simulink model "Final_project"  (R2015b)
settings: Solver=FixedStepDiscrete  StartTime=0.0  StopTime=10.0  RelTol=1e-3
InitFcn:
  | parameters
values from neighbouring files (symbols this model uses):
  Ak = 100    [parameters.m]
  b = 100    [parameters.m]
  dT = 0.01    [parameters.m]
  H = 20    [parameters.m]
  m = 2000    [parameters.m]
  pot_gain = .33    (= 0.33)    [parameters.m]
  pot_offset = 512    [parameters.m]
  R = 1/5    (= 0.2)    [parameters.m]
  V_Ki = 50    [parameters.m]
  V_Kp = 5000    [parameters.m]
undefined symbols (not defined in the file or in its folder): A10, A13, A14, AN0, AN12, B, B13, B4, B6, C6, D, D11, D4, DiscIntNeverNeededParam, F17, F3, F4, G4, H4, L3, PA10, PA11, PA12, PA13, PA14, PA5, PA6, PA7, PA8, PA9, PB10, PB7, PC6, PD10, PD11, PG4, R10, R16, R5, R8, T15
libraries: Conv_Lib x54, rappid_564xl_ec_toolbox x34, Veh_Sim x9, simulink x4, U_of_M_5643_blockset x1
(part 1 of 2)
settings Model: Creator=raoulkumar  LastModifiedBy=sutorimb
settings DataIOCC: ExternalInput=off  InitialState=off  SaveOutput=off  SignalLogging=off  SaveTime=off
settings OptimizationCC: DefaultParameterBehavior=Inlined  OptimizeModelRefInitCode=on  LifeSpan=1
settings DebuggingCC: InheritedTsInSrcMsg=none  SingleTaskRateTransMsg=error  UnconnectedInputMsg=error  UnconnectedOutputMsg=error  UnconnectedLineMsg=error  UnknownTsInhSupMsg=error
settings HardwareCC: ProdBitPerPointer=32  ProdLargestAtomicInteger=Long  ProdLargestAtomicFloat=Double  ProdEndianess=BigEndian  ProdWordSize=32  ProdHWDeviceType=Freescale->32-bit PowerPC
settings RTWCC: SystemTargetFile=rappid564xl.tlc  MakeCommand=rappid_564xl_make_rtw  TemplateMakefile=rappid_564xl_default_tmf  PostCodeGenCommand=rappid_analyzegencode(buildInfo)  Description=RAppID Toolbox MPC564xL Code Generation Target (rappid)  GenerateReport=on  IncludeHyperlinkInReport=on  LaunchReport=on  GenerateTraceReport=on  GenerateTraceReportSl=on  GenerateTraceReportSf=on  GenerateTraceReportEml=on
settings CodeAppCC: IgnoreCustomStorageClasses=off
settings STFCustomTargetCC: ConcurrentExecutionCompliant=off  GeneratePreprocessorConditionals=Use local settings  CombineOutputUpdateFcns=on  SuppressErrorStatus=on  ERTCustomFileBanners=on  SupportContinuousTime=off  SupportNonInlinedSFcns=off  MATLABClassNameForMDSCustomization=Simulink.SoftwareTarget.ERTCustomization  CPPClassGenCompliant=off  GRTInterface=off  SystemTargetFile=rappid564xl.tlc
settings ERTTargetCC: ParMdlRefBuildCompliant=off  CompOptLevelCompliant=off  ConcurrentExecutionCompliant=off  SuppressErrorStatus=on  ERTFirstTimeCompliant=off  ModelStepFunctionPrototypeControlCompliant=off  CPPClassGenCompliant=off  UseToolchainInfoCompliant=off  InlinedParameterPlacement=NonHierarchical  ERTCustomFileTemplate=example_file_process.tlc

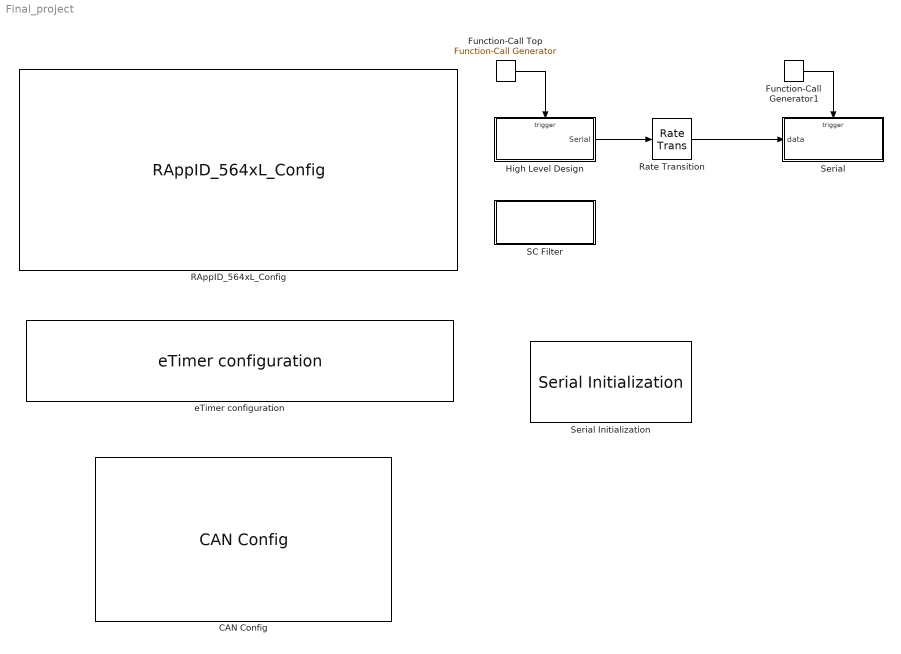
== system Final_project ==
  CAN Config : rappid_564xl_ec_toolbox/MPC564xL/Communication Blocks/CAN Config  Priority=1  can_unit=A  can_unit_v2=0  can_idam=A - One full ID (standard or extended) per filter element.  can_srx_dis=1 - Self reception disabled  can_presdiv=4  can_rjw=3  can_pseg1=5  can_pseg2=5  can_clk_src=0 - The CAN engine clock source is the oscillator clock  can_lpb=0 - Loop Back disabled  can_smp=0 - One sample is used to determine the bit value  can_boff_rec=0 - Automatic recovering from Bus Off state enabled  can_tsyn=0 - Timer Sync feature disabled  can_lbuf=0 - Buffer with highest priority is transmitted first  can_lom=0 - Listen Only Mode is deactivated  can_propseg=2
  Function-Call Generator1 : simulink/Ports & Subsystems/Function-Call Generator  sample_time=0.05  numberOfIterations=1
  Function-Call Top : simulink/Ports & Subsystems/Function-Call Generator  sample_time=dT  numberOfIterations=1
  High Level Design : Subsystem  TreatAsAtomicUnit=on
  RAppID_564xL_Config : rappid_564xl_ec_toolbox/MPC564xL/RAppID_564xL_Config  SystemClock=120  XTAL=40  MC_clock_60=12  MC_clock_80=16  MC_clock_120=10  SWG_clock_60=20  SWG_clock_80=13.334  SWG_clock_120=20  Compiler=CodeWarrior  MemTarget=FLASH  Part=MPC5643L  Package=144 LQFP  global_int_priority=10  base_tick_priority=11  sys_task_supress=off  exception_handlers=off  stored_mdl_name=Final_project  freemaster_interface=Oops  freemaster_rx_pin="LINFlex_0 Rx Pin 116 : \"PB[3]\""  freemaster_tx_pin="LINFlex_0 Tx Pin 114 : \"PB[2]\""  freemaster_interface_1=Serial 0  freemaster_enable=on  freemaster_rate=115200  freemaster_tx0_pin=18 : B[2] : 114 : A14  freemaster_rx0_pin=19 : B[3] : 116 : B13  freemaster_tx1_pin=57 : D[9] : 26 : L3  freemaster_rx1_pin=29 : B[13] : 60 : R10  freemaster_can_channel=1CH  freemater_can_speed=500K  freemaster_can_msgig=0x7AA  ccp_interface=None  ccp_enable=off  ccp_can_channel=CH1 (MB 0 - 1)  ccp_can_speed=500K  ccp_can_cro_id=256  ccp_can_dto_id=257  ccp_dev_id=RappID  ccp_dev_addr=0  ccp_odt=3  ccp_daq=3  pil_enable=off  pil_bam=off  comport=4  pil_rate=115200  bam_password_def=on  bam_password=0xFEEDFACECAFEBEEF  bam_sa_cs=off  bam_start_address=0x0  bam_code_size=0x7000  cons_dspi=on  cons_can=on  cons_adc=on  cons_pwm=on  cons_ctu=on  cons_swg=on  cons_eTimer=on  cons_fm=on
  Rate Transition : RateTransition
  SC Filter : Subsystem
  Serial : Subsystem  TreatAsAtomicUnit=on
  Serial Initialization : U_of_M_5643_blockset/Serial/Serial Initialization
  eTimer configuration : rappid_564xl_ec_toolbox/MPC564xL/Motor Control Blocks/eTimer configuration  SubModule=0  TimerChan=0  subMod=0  channel=0  CountMode=100 - Quadrature count mode using primary and secondary sources  CNTMODE=4  CountOnce=0 - Count repeatedly  ONCE=0  CountLength=0 - Continue counting to roll over  LENGTH=0  CountDirection=0 - Count up  DIR=0  OutputEnable=0 - The external pin is configured as an input  OEN=0  CoChanInit=00 - Other channels cannot force re-initialization of this channel  COINIT=0  StopAction=0 - Output enable is unaffected by stop mode  STPEN=0  ReloadOnCapt=00 - Do not reload the counter on a capture event  ROC=0  PrimarySource=00000 - Counter #0 input pin  PRISRC=0  PrimSrcPol=0 - True polarity  PIPS=0  SecondarySource=00001 - Counter #1 input pin  SECSRC=1  SecSrcPol=0 - True polarity  SIPS=0  FILT_CNT=0  FILT_PER=0  FILT=0  OutputMode=0000 - Software controlled  OUTMODE=0  OutputPol=0 - True polarity  OPS=0  MasterMode=0 - Disable broadcast of this channel output  MSTR=0  ForcedOutVal=0  VAL=0  CoForce=0 - Other channels cannot force this channel output  COFRC=0  CompLoad1=000 - COMP1 is never preload  CLC1=0  CompLoad2=000 - COMP2 is never preload  CLC2=0  CompareMode="00 - COMP1 and COMP2  are used when the counter is counting up"  CMPMODE=0  CaptMode1=00 - Capture disabled  CPT1MODE=0  CaptMode2=00 - Capture disabled  CPT2MODE=0  OneShCaptMode=0 - Free running mode is selected  ONESHOT=0  CaptFIFO=0  CFWM=0  CNTRinit=0  COMP1init=0  COMP2init=0  mod0ch0pin="0   : PA0  : [ 73 ] : [ T14 ]  input/output"  mod0ch1pin="1   : PA1  : [ 74 ] : [ R14 ]  input/output"  mod0ch2pin=None  mod0ch3pin=None  mod0ch4pin=None  mod0ch5pin=None  mod1ch0pin=None  mod1ch1pin=None  mod1ch2pin=None  mod1ch3pin=None  mod1ch4pin=None  mod1ch5pin=None  mod2ch0pin=None  mod2ch1pin=None  mod2ch2pin=None  mod2ch3pin=None  mod2ch4pin=None  mod2ch5pin=None  pcrNum0=0  pcrNum1=1  pcrNum2=255  pcrNum3=255  pcrNum4=255  pcrNum5=255  TCFIE=off  TCF1IE=off  TCF2IE=off  TOFIE=off  IELFIE=off  IEHFIE=off  ICF1IE=off  ICF2IE=off  INTDMA=0
  wires:
  Function-Call Top/1 -> High Level Design/Trigger
  Function-Call Generator1/1 -> Serial/Trigger
  High Level Design/1(Serial) -> Rate Transition/1
  Rate Transition/1 -> Serial/1(data)

== system Final_project/High Level Design ==
  function : TriggerPort  TriggerType=function-call
  "\tVehicle Model" : Subsystem
  Automatic Cruise Control : Subsystem
  Automatic Steering : Subsystem
  Delay : Delay  DelayLength=1  InitialCondition=0
  Inputs : Subsystem
  Outputs : Subsystem
  Terminator : Terminator
  Serial : Outport
  wires:
  Outputs/1("x, y, pxi (Cars 1-6)") -> Serial/1
  Inputs/3(Cruise Control Speed) -> Automatic Cruise Control/1(Cruise Control Speed)
  "\tVehicle Model"/1(s,n,psi us (This Car)) -> Automatic Steering/3("s, n, psi, us (This Car)"), Delay/1, Outputs/2("s, n, psi, us (This Car)")
  Inputs/2(ACC_enable) -> Automatic Cruise Control/2(Acc Enable)
  Inputs/6(Automatic Steering Enable) -> Automatic Steering/1(Automatic Steering Enable)
  Inputs/4(Steering Angle (delta)) -> "\tVehicle Model"/2(steering angle (delta)), Automatic Steering/2(Steering Angle (delta))
  Inputs/5(Throttle (Fd)) -> Automatic Cruise Control/5(Fd)
  "\tVehicle Model"/2(Self-Aligning Torque) -> Outputs/4(Self-Aligning Torque)
  Inputs/1("s, n, psi, us (Cars 1-6)") -> Automatic Cruise Control/3("s, n, psi, us (Cars 1-6)"), Outputs/1("s, n, psi, us (Cars 1-6)")
  "\tVehicle Model"/3(u) -> Outputs/3(u (This car))
  Automatic Steering/1(Auto Torque) -> Outputs/5(Auto Torque)
  Automatic Cruise Control/1(Fd_out) -> "\tVehicle Model"/1(Fd)
  Delay/1 -> Automatic Cruise Control/4(s,n,psi,us (This Car))
  Automatic Steering/2(delta_desired) -> Terminator/1

== system Final_project/SC Filter ==
  Constant1 : Constant  Value=1e6  OutDataTypeStr=uint32
  Constant2 : Constant  Value=0  OutDataTypeStr=uint32
  Constant3 : Constant  Value=50  OutDataTypeStr=uint32
  Simple PWM Output : rappid_564xl_ec_toolbox/MPC564xL/Motor Control Blocks/Simple PWM Output  Priority=1  pwmModule=0  pwmMod=0  SubModule=1  subMod=1  InitFreq=1000000  resolution=1 %  resValue=1  InitDutyA=0  InitDutyB=50  align=A B - edge aligned  PhaseShift_A=0  PhaseShift=0  Phase_A=0  Phase_B=0  centered=0  DoubleS=off  doubleSw=off  debugSw=off  debug_mode=0  pin_A0=None  pin_B0=None  pin_X0=None  pin_A1=None  pin_B1="38  : PC6  : [ 142 ] : [ D4 ]"  pin_X1=None  pin_A2=None  pin_B2=None  pin_X2=None  pin_A3=None  pin_B3=None  pin_X3=None  pin1_A0=None  pin1_B0=None  pin1_X0=None  pin1_A1=None  pin1_B1=None  pin1_X1=None  pin1_A2=None  pin1_B2=None  pin1_X2=None  pin1_A3=None  pin1_B3=None  pin1_X3=None  pcrNumA=255  pcrNumB=38  pcrNumX=255  polA=off  polB=off  polX=off  octrl=0  syncFrom0=off  masterSync=0  outVal0=off  outVal1=off  outVal2=off  outVal3=off  outVal4=on  outVal5=on  outTrig=48
  wires:
  Constant1/1 -> Simple PWM Output/1
  Constant2/1 -> Simple PWM Output/2
  Constant3/1 -> Simple PWM Output/3

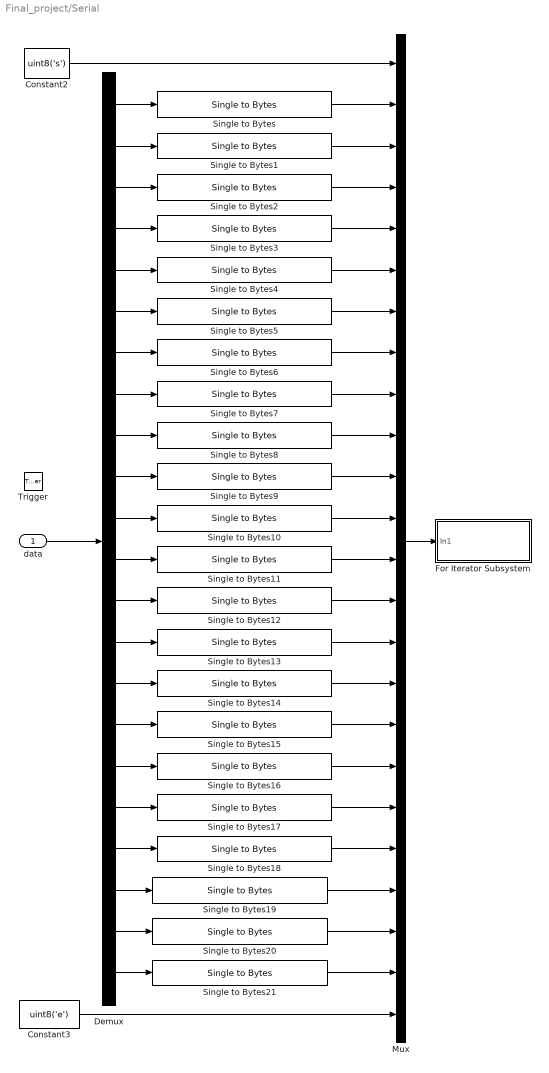
== system Final_project/Serial ==
  data : Inport
  Trigger : TriggerPort  TriggerType=function-call
  Constant2 : Constant  Value=uint8('s')  OutDataTypeStr=uint8
  Constant3 : Constant  Value=uint8('e')  OutDataTypeStr=uint8
  Demux : Demux  Outputs=22
  For Iterator Subsystem : Subsystem
  Mux : Mux  Inputs=24
  Single to Bytes{,1..21} (22 alike) : Conv_Lib/Single to Bytes
  wires:
  Constant2/1 -> Mux/1
  Single to Bytes/1 -> Mux/2
  Single to Bytes1/1 -> Mux/3
  Single to Bytes2/1 -> Mux/4
  Single to Bytes3/1 -> Mux/5
  Single to Bytes4/1 -> Mux/6
  Single to Bytes5/1 -> Mux/7
  Single to Bytes6/1 -> Mux/8
  Single to Bytes7/1 -> Mux/9
  Single to Bytes8/1 -> Mux/10
  Single to Bytes9/1 -> Mux/11
  Single to Bytes10/1 -> Mux/12
  Single to Bytes11/1 -> Mux/13
  Single to Bytes12/1 -> Mux/14
  Single to Bytes13/1 -> Mux/15
  Single to Bytes15/1 -> Mux/17
  Single to Bytes16/1 -> Mux/18
  Single to Bytes17/1 -> Mux/19
  Mux/1 -> For Iterator Subsystem/1(In1)
  Demux/1 -> Single to Bytes/1
  Demux/2 -> Single to Bytes1/1
  Demux/3 -> Single to Bytes2/1
  Demux/4 -> Single to Bytes3/1
  Demux/5 -> Single to Bytes4/1
  Demux/6 -> Single to Bytes5/1
  Demux/7 -> Single to Bytes6/1
  Demux/8 -> Single to Bytes7/1
  Demux/9 -> Single to Bytes8/1
  Demux/10 -> Single to Bytes9/1
  Demux/11 -> Single to Bytes10/1
  Demux/12 -> Single to Bytes11/1
  Demux/13 -> Single to Bytes12/1
  Demux/14 -> Single to Bytes13/1
  Demux/15 -> Single to Bytes14/1
  Demux/16 -> Single to Bytes15/1
  Demux/17 -> Single to Bytes16/1
  Demux/18 -> Single to Bytes17/1
  data/1 -> Demux/1
  Single to Bytes14/1 -> Mux/16
  Demux/19 -> Single to Bytes18/1
  Demux/20 -> Single to Bytes19/1
  Demux/21 -> Single to Bytes20/1
  Demux/22 -> Single to Bytes21/1
  Single to Bytes18/1 -> Mux/20
  Single to Bytes19/1 -> Mux/21
  Single to Bytes20/1 -> Mux/22
  Single to Bytes21/1 -> Mux/23
  Constant3/1 -> Mux/24

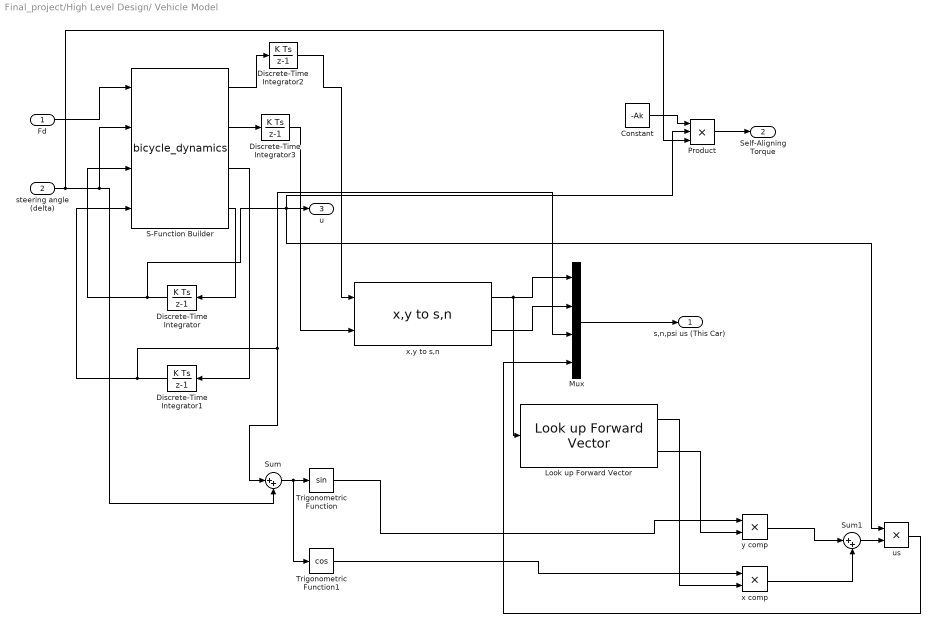
== system Final_project/High Level Design/	Vehicle Model ==
  Fd : Inport
  steering angle (delta) : Inport  Port=2
  Constant : Constant  Value=-Ak  OutDataTypeStr=single
  Discrete-Time Integrator{,1..3} (4 alike) : DiscreteIntegrator  SampleTime=-1  ICPrevOutput=DiscIntNeverNeededParam  ICPrevScaledInput=DiscIntNeverNeededParam
  Look up Forward Vector : Veh_Sim/Look up Forward Vector  SystemSampleTime=-1
  Mux : Mux
  Product : Product  Inputs=3
  S-Function Builder : S-Function  InitFcn=try, set_param(gcb,'FunctionName','bicycle_dynamics'), end  FunctionName=bicycle_dynamics  SFunctionModules=bicycle_dynamics_wrapper  SFunctionDeploymentMode=off  EnableBusSupport=off  mask(S-Function Builder){}
      mask help: Simulink:masks:SFunctionBuilder_MD
      mask init:
      | val = [[.9  0.75 0.75 1 1 .9 .9 1]',[1 1 0.75 0.75 .9 .9 1 .9]'];try , sys = get_param(gcb,'SfunBuilderFcnName');if isempty(sys), sys = get_param(gcb,'FunctionName'); end,catch, sys = get_param(gcb,'FunctionName'); end
      settings: CopyFcn=set_param(gcbh,'LinkStatus','none')  PreSaveFcn=try, set_param(gcb,'FunctionName','bicycle_dynamics'), end  OpenFcn=sfunctionwizard(gcbh)
      mask Display: plot(val(:,1),val(:,2)),disp(sys), port_label('input',1,'Fd'), port_label('input',2,'delta'), port_label('input',3,'u'), port_label('input',4,'psi'), port_label('output',1,'x_dot'), port_label('output',2,'y_dot'), port_label('output',3,'psi_dot'), port_label('output',4,'u_dot')
  Sum : Sum  Inputs=|++
  Sum1 : Sum  Inputs=|++
  Trigonometric Function : Trigonometry
  Trigonometric Function1 : Trigonometry  Operator=cos
  "us " : Product
  x comp : Product
  x,y to s,n : Veh_Sim/x,y to s,n  SystemSampleTime=-1
  y comp : Product
  s,n,psi us (This Car) : Outport
  Self-Aligning Torque : Outport  Port=2
  u : Outport  Port=3
  wires:
  Fd/1 -> S-Function Builder/1
  steering angle (delta)/1 -> Product/3, Sum/2, S-Function Builder/2
  S-Function Builder/4 -> Discrete-Time Integrator/1
  S-Function Builder/3 -> Discrete-Time Integrator1/1
  Discrete-Time Integrator/1 -> "us "/1, Product/2, u/1, S-Function Builder/3
  Discrete-Time Integrator1/1 -> Mux/3, Sum/1, S-Function Builder/4
  S-Function Builder/1 -> Discrete-Time Integrator2/1
  Discrete-Time Integrator2/1 -> x,y to s,n/1
  Discrete-Time Integrator3/1 -> x,y to s,n/2
  S-Function Builder/2 -> Discrete-Time Integrator3/1
  Constant/1 -> Product/1
  Product/1 -> Self-Aligning Torque/1
  Mux/1 -> s,n,psi us (This Car)/1
  x,y to s,n/1 -> Look up Forward Vector/1, Mux/1
  x,y to s,n/2 -> Mux/2
  Sum/1 -> Trigonometric Function1/1, Trigonometric Function/1
  Trigonometric Function/1 -> y comp/1
  Look up Forward Vector/2 -> y comp/2
  Trigonometric Function1/1 -> x comp/1
  Look up Forward Vector/1 -> x comp/2
  y comp/1 -> Sum1/1
  x comp/1 -> Sum1/2
  Sum1/1 -> "us "/2
  "us "/1 -> Mux/4

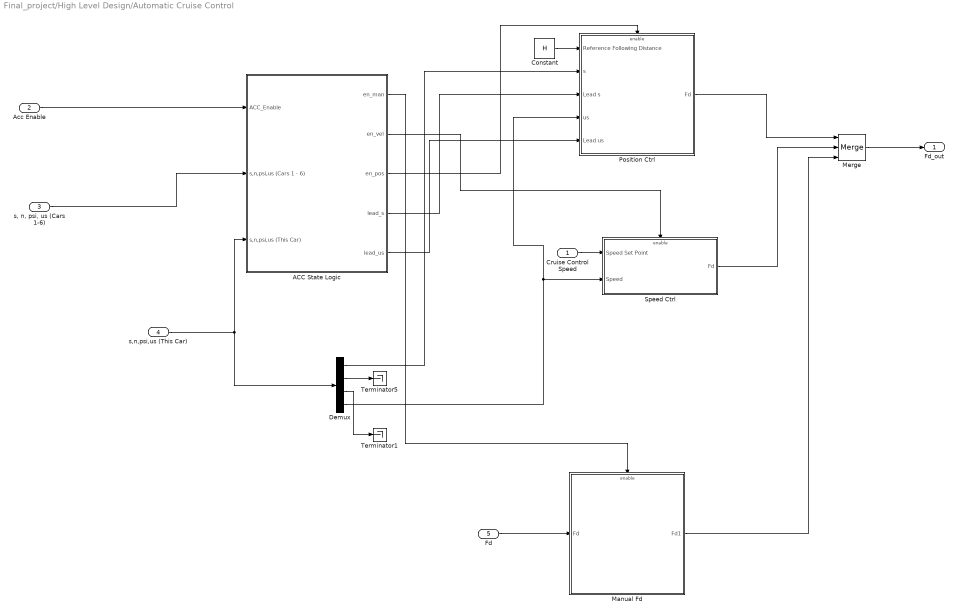
== system Final_project/High Level Design/Automatic Cruise Control ==
  Cruise Control Speed : Inport
  Acc Enable : Inport  Port=2
  "s, n, psi, us (Cars 1-6)" : Inport  Port=3
  s,n,psi,us (This Car) : Inport  Port=4
  Fd : Inport  Port=5
  ACC State Logic : Subsystem
  Constant : Constant  Value=H
  Demux : Demux
  Manual Fd : Subsystem  TreatAsAtomicUnit=on
  Merge : Merge  Inputs=3
  Position Ctrl : Subsystem  TreatAsAtomicUnit=on
  Speed Ctrl : Subsystem  TreatAsAtomicUnit=on
  Terminator1 : Terminator
  Terminator5 : Terminator
  Fd_out : Outport
  wires:
  Acc Enable/1 -> ACC State Logic/1(ACC_Enable)
  "s, n, psi, us (Cars 1-6)"/1 -> ACC State Logic/2(s,n,psi,us (Cars 1 - 6))
  s,n,psi,us (This Car)/1 -> Demux/1, ACC State Logic/3(s,n,psi,us (This Car))
  ACC State Logic/3(en_pos) -> Position Ctrl/Enable
  ACC State Logic/2(en_vel) -> Speed Ctrl/Enable
  ACC State Logic/4(lead_s) -> Position Ctrl/3(Lead s)
  Cruise Control Speed/1 -> Speed Ctrl/1(Speed Set Point)
  ACC State Logic/5(lead_us) -> Position Ctrl/5(Lead us)
  Demux/1 -> Position Ctrl/2(s)
  Demux/4 -> Position Ctrl/4(us), Speed Ctrl/2(Speed)
  Position Ctrl/1(Fd) -> Merge/1
  Speed Ctrl/1(Fd) -> Merge/2
  Constant/1 -> Position Ctrl/1(Reference Following Distance)
  Fd/1 -> Manual Fd/1(Fd)
  Manual Fd/1(Fd1) -> Merge/3
  ACC State Logic/1(en_man) -> Manual Fd/Enable
  Merge/1 -> Fd_out/1
  Demux/2 -> Terminator5/1
  Demux/3 -> Terminator1/1

== system Final_project/High Level Design/Automatic Steering ==
  Automatic Steering Enable : Inport
  Steering Angle (delta) : Inport  Port=2
  "s, n, psi, us (This Car)" : Inport  Port=3
  Constant : Constant  Value=0.5  OutDataTypeStr=single
  Controller : Subsystem  TreatAsAtomicUnit=on
  Demux : Demux
  Terminator : Terminator
  Terminator1 : Terminator
  Terminator3 : Terminator
  Auto Torque : Outport
  delta_desired : Outport  Port=2
  wires:
  Automatic Steering Enable/1 -> Controller/Enable
  Controller/1(Auto Torque) -> Auto Torque/1
  "s, n, psi, us (This Car)"/1 -> Demux/1
  Demux/4 -> Terminator/1
  Demux/3 -> Terminator1/1
  Demux/1 -> Terminator3/1
  Demux/2 -> Controller/1(n (This Car))
  Steering Angle (delta)/1 -> Controller/3(Delta (This Car))
  Constant/1 -> Controller/2(n desired)
  Controller/2(delta desired) -> delta_desired/1

== system Final_project/High Level Design/Inputs ==
  Digital Input : rappid_564xl_ec_toolbox/MPC564xL/General Purpose Blocks/Digital Input  gpio_outputs="13  : PA13 : [ 136 ] : [ C6 ]"  pinNum=[ 136 ]  pcrNum=13
  Digital Input1 : rappid_564xl_ec_toolbox/MPC564xL/General Purpose Blocks/Digital Input  gpio_outputs="14  : PA14 : [ 143 ] : [ B4 ]"  pinNum=[ 143 ]  pcrNum=14
  Gain : Gain  Gain=R/10
  Other Cars : Subsystem
  Select Speed (GPI 122-129) : Subsystem
  Throttle (Potentiometer) : Subsystem
  get wheel position : Subsystem
  "s, n, psi, us (Cars 1-6)" : Outport
  ACC_enable : Outport  Port=2
  Cruise Control Speed : Outport  Port=3
  Steering Angle (delta) : Outport  Port=4
  Throttle (Fd) : Outport  Port=5
  Automatic Steering Enable : Outport  Port=6
  wires:
  Other Cars/1("s, n, psi, us (Cars 1-6)") -> "s, n, psi, us (Cars 1-6)"/1
  Select Speed (GPI 122-129)/1(Speed) -> Cruise Control Speed/1
  get wheel position/1(Haptic Wheel Position (radians)) -> Gain/1
  Gain/1 -> Steering Angle (delta)/1
  Throttle (Potentiometer)/1(Fd) -> Throttle (Fd)/1
  Digital Input/1 -> ACC_enable/1
  Digital Input1/1 -> Automatic Steering Enable/1

== system Final_project/High Level Design/Outputs ==
  "s, n, psi, us (Cars 1-6)" : Inport
  "s, n, psi, us (This Car)" : Inport  Port=2
  u (This car) : Inport  Port=3
  Self-Aligning Torque : Inport  Port=4
  Auto Torque : Inport  Port=5
  Extract x,y,psi : Subsystem
  Extract x,y,psi (Cars 1 - 6) : Subsystem
  Mux : Mux  Inputs=3
  Output s,n,psi,us : Subsystem
  Sum1 : Sum  Inputs=|++
  write torque : Subsystem
  "x, y, pxi (Cars 1-6)" : Outport
  wires:
  Self-Aligning Torque/1 -> Sum1/1
  Auto Torque/1 -> Sum1/2
  Sum1/1 -> write torque/1(Reaction Torque)
  "s, n, psi, us (Cars 1-6)"/1 -> Extract x,y,psi (Cars 1 - 6)/1(s,n,psi,us (Cars 1 - 6))
  "s, n, psi, us (This Car)"/1 -> Output s,n,psi,us/1(s,n,psi.us), Extract x,y,psi/1(s,n,psi,us)
  Extract x,y,psi/1(x,y,psi) -> Mux/1
  Mux/1 -> "x, y, pxi (Cars 1-6)"/1
  u (This car)/1 -> Mux/2
  Extract x,y,psi (Cars 1 - 6)/1(x,y,psi (Cars 1 - 6)) -> Mux/3

== system Final_project/Serial/For Iterator Subsystem ==
  In1 : Inport
  Data Type Conversion : DataTypeConversion  OutDataTypeStr=uint8
  For Iterator : ForIterator  IterationLimit=90  IndexMode=Zero-based  IterationVariableDataType=int8
  Index Vector : MultiPortSwitch  DataPortOrder=Zero-based contiguous  Inputs=1  zeroidx=on
  S-Function : S-Function  FunctionName=SerialSend  SFunctionDeploymentMode=off  EnableBusSupport=off
      mask Display:
      | patch([0 0 1 1], [0 1 1 0], [255/255 255/255 0])
      | patch([0 0 0.05 0.05], [0 1 1 0], [0 0 255/255])
      | patch([1 1 0.95 0.95], [0 1 1 0], [0 0 255/255])
      | 
      | text (0.52, 0.8, ['Serial Send'], 'horizontalAlignment', 'center');
      | %text (0.5, .5, ['System Clock MHz: ' get_param(gcb,'SystemClock')], 'horizontalAlignment', 'center');
      | %text (0.5, .35, ['Baud Rate: ' get_param(gcb,'BaudRate')], 'horizontalAlignment', 'center');
      | text(0.5, 0.1, 'The University of Michigan', 'horizontalAlignment', 'center');
  wires:
  In1/1 -> Index Vector/2
  Index Vector/1 -> Data Type Conversion/1
  For Iterator/1 -> Index Vector/1
  Data Type Conversion/1 -> S-Function/1

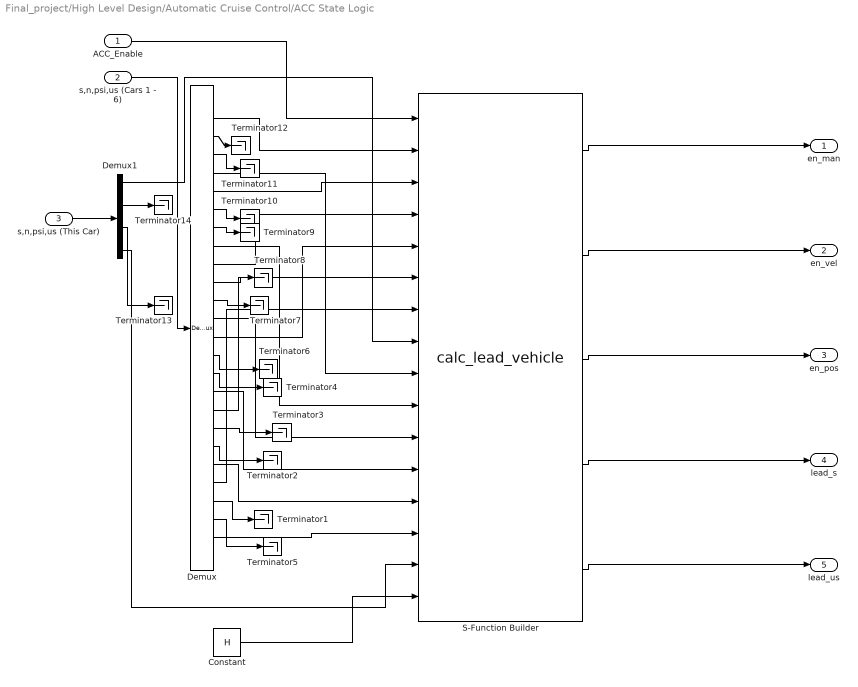
== system Final_project/High Level Design/Automatic Cruise Control/ACC State Logic ==
  ACC_Enable : Inport
  s,n,psi,us (Cars 1 - 6) : Inport  Port=2
  s,n,psi,us (This Car) : Inport  Port=3
  Constant : Constant  Value=H
  Demux : Demux  Outputs=24
  Demux1 : Demux
  S-Function Builder : S-Function  InitFcn=try, set_param(gcb,'FunctionName','calc_lead_vehicle'), end  FunctionName=calc_lead_vehicle  SFunctionModules=calc_lead_vehicle_wrapper  SFunctionDeploymentMode=off  EnableBusSupport=off  mask(S-Function Builder){}
      mask help: Simulink:masks:SFunctionBuilder_MD
      mask init: same as Final_project/High Level Design/	Vehicle Model/S-Function Builder
      settings: CopyFcn=set_param(gcbh,'LinkStatus','none')  PreSaveFcn=try, set_param(gcb,'FunctionName','calc_lead_vehicle'), end  OpenFcn=sfunctionwizard(gcbh)
      mask Display: plot(val(:,1),val(:,2)),disp(sys), port_label('input',1,'ACC_Enable'), port_label('input',2,'s1'), port_label('input',3,'s2'), port_label('input',4,'s3'), port_label('input',5,'s4'), port_label('input',6,'s5'), port_label('input',7,'s6'), port_label('input',8,'s'), port_label('input',9,'us1'), port_label('input',10,'us2'), port_label('input',11,'us3'), port_label('input',12,'us4'), port_label('input',13,'us5'), port_label('input',14,'us6'), port_label('input',15,'us'), port_label('input',16,'H'), port_label('output',1,'en_man'), port_label('output',2,'en_vel'), port_label('output',3,'en_pos'), port_label('output',4,'lead_s'), port_label('output',5,'lead_us')
  Terminator{1..14} (14 alike) : Terminator
  en_man : Outport
  en_vel : Outport  Port=2
  en_pos : Outport  Port=3
  lead_s : Outport  Port=4
  lead_us : Outport  Port=5
  wires:
  s,n,psi,us (Cars 1 - 6)/1 -> Demux/1
  s,n,psi,us (This Car)/1 -> Demux1/1
  ACC_Enable/1 -> S-Function Builder/1
  S-Function Builder/1 -> en_man/1
  S-Function Builder/2 -> en_vel/1
  S-Function Builder/3 -> en_pos/1
  S-Function Builder/4 -> lead_s/1
  S-Function Builder/5 -> lead_us/1
  Constant/1 -> S-Function Builder/16
  Demux1/4 -> S-Function Builder/15
  Demux/1 -> S-Function Builder/2
  Demux/4 -> S-Function Builder/9
  Demux/5 -> S-Function Builder/3
  Demux/8 -> S-Function Builder/10
  Demux/9 -> S-Function Builder/4
  Demux/12 -> S-Function Builder/11
  Demux/13 -> S-Function Builder/5
  Demux/16 -> S-Function Builder/12
  Demux/17 -> S-Function Builder/6
  Demux/20 -> S-Function Builder/13
  Demux/24 -> S-Function Builder/14
  Demux/21 -> S-Function Builder/7
  Demux1/1 -> S-Function Builder/8
  Demux/23 -> Terminator5/1
  Demux/22 -> Terminator1/1
  Demux/19 -> Terminator2/1
  Demux/18 -> Terminator3/1
  Demux/15 -> Terminator4/1
  Demux/14 -> Terminator6/1
  Demux/11 -> Terminator7/1
  Demux/10 -> Terminator8/1
  Demux/7 -> Terminator9/1
  Demux/6 -> Terminator10/1
  Demux/3 -> Terminator11/1
  Demux/2 -> Terminator12/1
  Demux1/3 -> Terminator13/1
  Demux1/2 -> Terminator14/1

== system Final_project/High Level Design/Automatic Cruise Control/Manual Fd ==
  Fd : Inport
  Enable : EnablePort
  Fd1 : Outport
  wires:
  Fd/1 -> Fd1/1

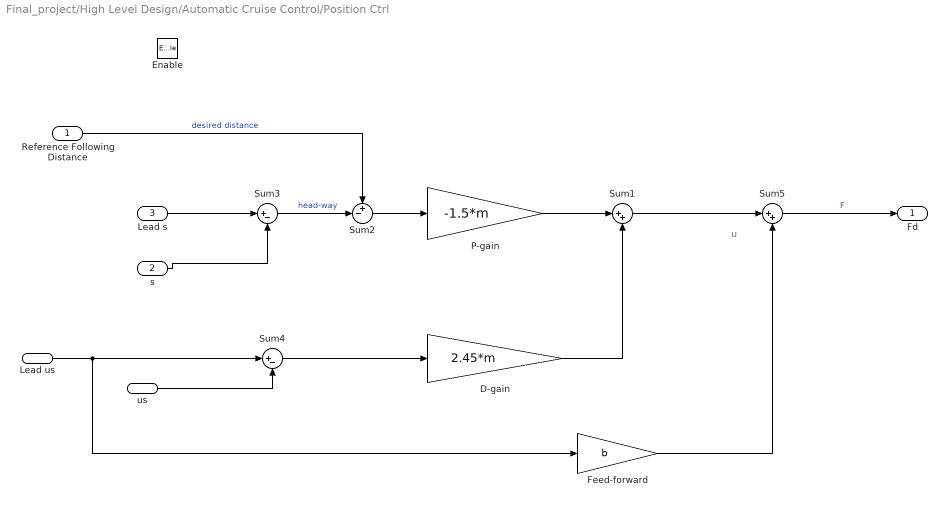
== system Final_project/High Level Design/Automatic Cruise Control/Position Ctrl ==
  note: u
  Reference Following Distance : Inport
  s : Inport  Port=2
  Lead s : Inport  Port=3
  us : Inport  Port=4
  Lead us : Inport  Port=5
  Enable : EnablePort
  D-gain : Gain  Gain=2.45*m  SaturateOnIntegerOverflow=on  OutDataTypeStr=Inherit: Same as input  ParamDataTypeStr=Inherit: Same as input
  Feed-forward : Gain  Gain=b  SaturateOnIntegerOverflow=on  OutDataTypeStr=Inherit: Same as input  ParamDataTypeStr=Inherit: Same as input
  P-gain : Gain  Gain=-1.5*m  SaturateOnIntegerOverflow=on  OutDataTypeStr=Inherit: Same as input  ParamDataTypeStr=Inherit: Same as input
  Sum1 : Sum  Inputs=|++  SaturateOnIntegerOverflow=on
  Sum2 : Sum  Inputs=+-|  SaturateOnIntegerOverflow=on
  Sum3 : Sum  Inputs=|+-  SaturateOnIntegerOverflow=on
  Sum4 : Sum  Inputs=|+-  SaturateOnIntegerOverflow=on
  Sum5 : Sum  Inputs=|++  OutDataTypeStr=single  SaturateOnIntegerOverflow=on
  Fd : Outport
  wires:
  Lead s/1 -> Sum3/1
  s/1 -> Sum3/2
  Reference Following Distance/1 -> Sum2/1  "desired distance"
  Sum3/1 -> Sum2/2  "head-way"
  Sum2/1 -> P-gain/1
  P-gain/1 -> Sum1/1
  D-gain/1 -> Sum1/2
  us/1 -> Sum4/2
  Lead us/1 -> Sum4/1, Feed-forward/1
  Sum4/1 -> D-gain/1
  Feed-forward/1 -> Sum5/2
  Sum5/1 -> Fd/1  "F"
  Sum1/1 -> Sum5/1

== system Final_project/High Level Design/Automatic Cruise Control/Speed Ctrl ==
  Speed Set Point : Inport
  Speed : Inport  Port=2
  Enable : EnablePort
  Gain : Gain  Gain=b  SaturateOnIntegerOverflow=on  OutDataTypeStr=Inherit: Same as input  ParamDataTypeStr=Inherit: Same as input
  PI : Subsystem
  Sum : Sum  Inputs=++|  OutDataTypeStr=single  SaturateOnIntegerOverflow=on
  Sum1 : Sum  Inputs=|+-  SaturateOnIntegerOverflow=on
  Fd : Outport
  wires:
  Sum/1 -> Fd/1  "Fd"
  Speed Set Point/1 -> Gain/1, Sum1/1  "desired speed"
  Speed/1 -> Sum1/2
  Sum1/1 -> PI/1(Error)
  Gain/1 -> Sum/1
  PI/1(U) -> Sum/2

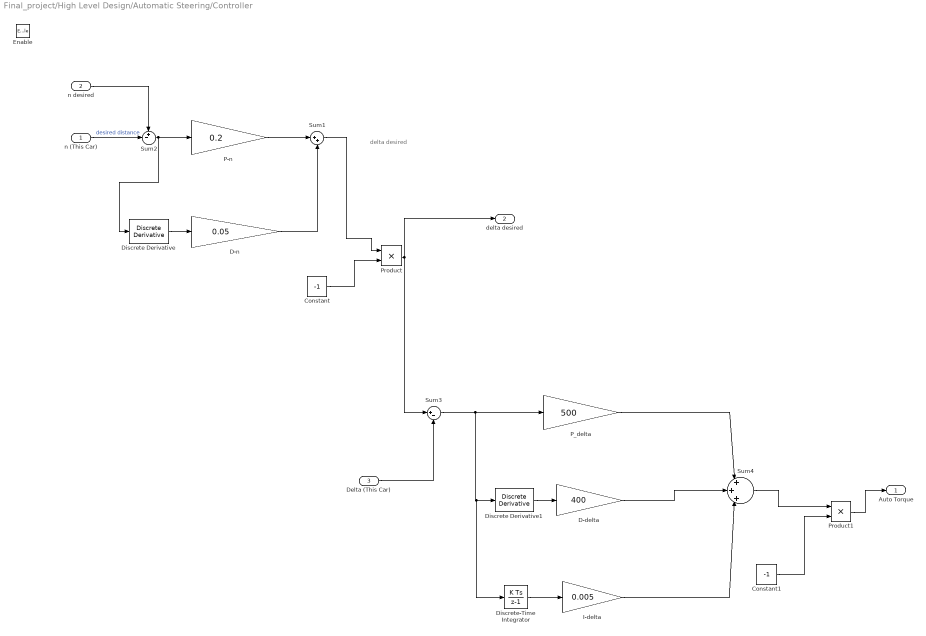
== system Final_project/High Level Design/Automatic Steering/Controller ==
  note: delta desired
  n (This Car) : Inport
  n desired : Inport  Port=2
  Delta (This Car) : Inport  Port=3
  Enable : EnablePort
  Constant : Constant  Value=-1  OutDataTypeStr=single
  Constant1 : Constant  Value=-1  OutDataTypeStr=single
  D-delta : Gain  Gain=400  SaturateOnIntegerOverflow=on  OutDataTypeStr=Inherit: Same as input  ParamDataTypeStr=Inherit: Same as input
  D-n : Gain  Gain=0.05  SaturateOnIntegerOverflow=on  OutDataTypeStr=Inherit: Same as input  ParamDataTypeStr=Inherit: Same as input
  Discrete Derivative : simulink/Discrete/Discrete Derivative  gainval=1.0  ICPrevScaledInput=0.0  InputProcessing=Inherited  OutMin=[]  OutMax=[]  OutDataTypeStr=single  OutputDataTypeScalingMode=single  OutDataType=fixdt(1, 16)  OutScaling=2^-10  DoSatur=off
  Discrete Derivative1 : simulink/Discrete/Discrete Derivative  gainval=1.0  ICPrevScaledInput=0.0  InputProcessing=Inherited  OutMin=[]  OutMax=[]  OutDataTypeStr=single  OutputDataTypeScalingMode=single  OutDataType=fixdt(1, 16)  OutScaling=2^-10  DoSatur=off
  Discrete-Time Integrator : DiscreteIntegrator  SampleTime=-1  ICPrevOutput=DiscIntNeverNeededParam  ICPrevScaledInput=DiscIntNeverNeededParam
  I-delta : Gain  Gain=0.005  SaturateOnIntegerOverflow=on  OutDataTypeStr=Inherit: Same as input  ParamDataTypeStr=Inherit: Same as input
  P-n : Gain  Gain=0.2  SaturateOnIntegerOverflow=on  OutDataTypeStr=Inherit: Same as input  ParamDataTypeStr=Inherit: Same as input
  P_delta : Gain  Gain=500  SaturateOnIntegerOverflow=on  OutDataTypeStr=Inherit: Same as input  ParamDataTypeStr=Inherit: Same as input
  Product : Product  OutDataTypeStr=single
  Product1 : Product  OutDataTypeStr=single
  Sum1 : Sum  Inputs=|++  SaturateOnIntegerOverflow=on
  Sum2 : Sum  Inputs=+-|  SaturateOnIntegerOverflow=on
  Sum3 : Sum  Inputs=|+-  SaturateOnIntegerOverflow=on
  Sum4 : Sum  Inputs=|+|+|+|  SaturateOnIntegerOverflow=on
  Auto Torque : Outport
  delta desired : Outport  Port=2
  wires:
  n desired/1 -> Sum2/1
  Sum2/1 -> P-n/1, Discrete Derivative/1
  P-n/1 -> Sum1/1
  D-n/1 -> Sum1/2
  Sum1/1 -> Product/1
  n (This Car)/1 -> Sum2/2  "desired distance"
  Discrete Derivative/1 -> D-n/1
  Delta (This Car)/1 -> Sum3/2
  Sum3/1 -> Discrete-Time Integrator/1, Discrete Derivative1/1, P_delta/1
  Discrete Derivative1/1 -> D-delta/1
  Discrete-Time Integrator/1 -> I-delta/1
  I-delta/1 -> Sum4/3
  D-delta/1 -> Sum4/2
  P_delta/1 -> Sum4/1
  Constant/1 -> Product/2
  Product/1 -> Sum3/1, delta desired/1
  Constant1/1 -> Product1/2
  Sum4/1 -> Product1/1
  Product1/1 -> Auto Torque/1

== system Final_project/High Level Design/Inputs/Other Cars ==
  " Car1" : Subsystem
  "1 for GSI vehicle only, 0 for ALL student vehicles fixed 4/16" : Constant
  Cars 2-5 : Subsystem
  GSI Car : Subsystem
  Mux1 : Mux  Inputs=2
  Mux2 : Mux  Inputs=2
  Switch : Switch  Criteria=u2 ~= 0
  Zeros (16) : Subsystem
  "s, n, psi, us (Cars 1-6)" : Outport
  wires:
  GSI Car/1(s,n,psi,us) -> Mux1/1
  Zeros (16)/1(Zeros) -> Mux1/2
  Mux1/1 -> Switch/1
  Switch/1 -> "s, n, psi, us (Cars 1-6)"/1
  "1 for GSI vehicle only, 0 for ALL student vehicles fixed 4/16"/1 -> Switch/2
  " Car1"/1(s,n,psi,us) -> Mux2/1
  Cars 2-5/1(s,n,psi,us) -> Mux2/2
  Mux2/1 -> Switch/3

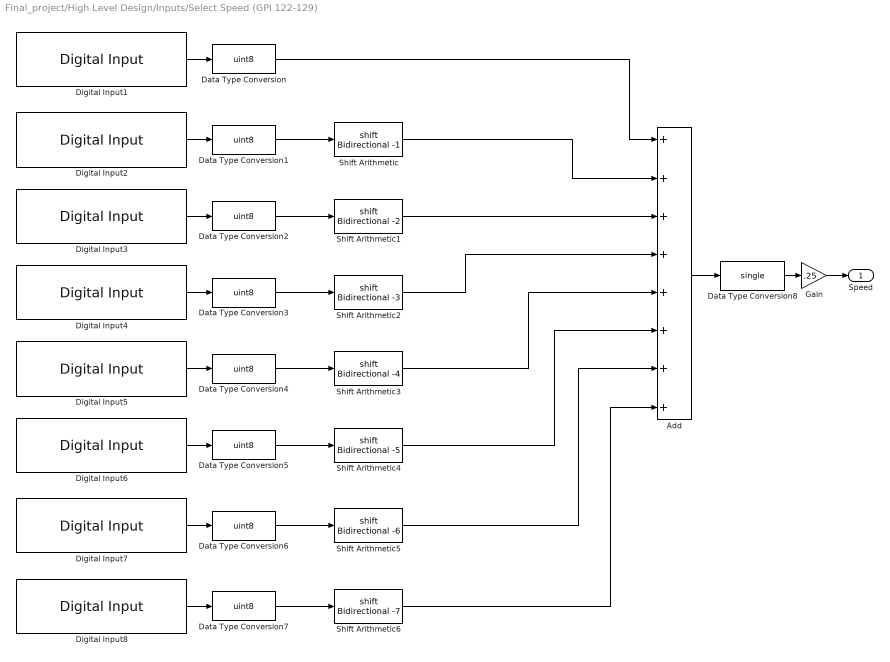
== system Final_project/High Level Design/Inputs/Select Speed (GPI 122-129) ==
  Add : Sum  Inputs=++++++++
  Data Type Conversion{,1..7} (8 alike) : DataTypeConversion  OutDataTypeStr=uint8
  Data Type Conversion8 : DataTypeConversion  OutDataTypeStr=single
  Digital Input1 : rappid_564xl_ec_toolbox/MPC564xL/General Purpose Blocks/Digital Input  gpio_outputs="5   : PA5  : [ 14 ] : [ H4 ]"  pinNum=[ 14 ]  pcrNum=5
  Digital Input2 : rappid_564xl_ec_toolbox/MPC564xL/General Purpose Blocks/Digital Input  gpio_outputs="6   : PA6  : [ 2 ] : [ G4 ]"  pinNum=[ 2 ]  pcrNum=6
  Digital Input3 : rappid_564xl_ec_toolbox/MPC564xL/General Purpose Blocks/Digital Input  gpio_outputs="7   : PA7  : [ 10 ] : [ F3 ]"  pinNum=[ 10 ]  pcrNum=7
  Digital Input4 : rappid_564xl_ec_toolbox/MPC564xL/General Purpose Blocks/Digital Input  gpio_outputs="8   : PA8  : [ 12 ] : [ F4 ]"  pinNum=[ 12 ]  pcrNum=8
  Digital Input5 : rappid_564xl_ec_toolbox/MPC564xL/General Purpose Blocks/Digital Input  gpio_outputs="9   : PA9  : [ 134 ] : [ B6 ]"  pinNum=[ 134 ]  pcrNum=9
  Digital Input6 : rappid_564xl_ec_toolbox/MPC564xL/General Purpose Blocks/Digital Input  gpio_outputs="10  : PA10  : [ 118 ] : [ A13 ]"  pinNum=[ 118 ]  pcrNum=10
  Digital Input7 : rappid_564xl_ec_toolbox/MPC564xL/General Purpose Blocks/Digital Input  gpio_outputs="11  : PA11 : [ 120 ] : [ D11 ]"  pinNum=[ 120 ]  pcrNum=11
  Digital Input8 : rappid_564xl_ec_toolbox/MPC564xL/General Purpose Blocks/Digital Input  gpio_outputs="12  : PA12 : [ 122 ] : [ A10 ]"  pinNum=[ 122 ]  pcrNum=12
  Gain : Gain  Gain=.25
  Shift Arithmetic : ArithShift  BitShiftNumber=-1
  Shift Arithmetic1 : ArithShift  BitShiftNumber=-2
  Shift Arithmetic2 : ArithShift  BitShiftNumber=-3
  Shift Arithmetic3 : ArithShift  BitShiftNumber=-4
  Shift Arithmetic4 : ArithShift  BitShiftNumber=-5
  Shift Arithmetic5 : ArithShift  BitShiftNumber=-6
  Shift Arithmetic6 : ArithShift  BitShiftNumber=-7
  Speed : Outport
  wires:
  Data Type Conversion1/1 -> Shift Arithmetic/1
  Data Type Conversion2/1 -> Shift Arithmetic1/1
  Data Type Conversion3/1 -> Shift Arithmetic2/1
  Data Type Conversion4/1 -> Shift Arithmetic3/1
  Data Type Conversion5/1 -> Shift Arithmetic4/1
  Data Type Conversion6/1 -> Shift Arithmetic5/1
  Data Type Conversion7/1 -> Shift Arithmetic6/1
  Data Type Conversion/1 -> Add/1
  Shift Arithmetic/1 -> Add/2
  Shift Arithmetic1/1 -> Add/3
  Shift Arithmetic2/1 -> Add/4
  Shift Arithmetic3/1 -> Add/5
  Shift Arithmetic4/1 -> Add/6
  Shift Arithmetic5/1 -> Add/7
  Shift Arithmetic6/1 -> Add/8
  Add/1 -> Data Type Conversion8/1
  Data Type Conversion8/1 -> Gain/1
  Gain/1 -> Speed/1
  Digital Input1/1 -> Data Type Conversion/1
  Digital Input2/1 -> Data Type Conversion1/1
  Digital Input3/1 -> Data Type Conversion2/1
  Digital Input4/1 -> Data Type Conversion3/1
  Digital Input5/1 -> Data Type Conversion4/1
  Digital Input6/1 -> Data Type Conversion5/1
  Digital Input7/1 -> Data Type Conversion6/1
  Digital Input8/1 -> Data Type Conversion7/1

== system Final_project/High Level Design/Inputs/Throttle (Potentiometer) ==
  ADC Channel : rappid_564xl_ec_toolbox/MPC564xL/Motor Control Blocks/ADC Channel  adc_unit=0  adc_chan0=older  adc_chan0_v2=23 : PB7 : [43] : [R5] : AN0  adc_chan1=older  adc_chan1_v2=26 : PB10 : [53] : [R8] : AN12  simulate=off  interrupt=off  adc_mode=Normal  adc_presample=off
  ADC Config : rappid_564xl_ec_toolbox/MPC564xL/Motor Control Blocks/ADC Config  adc_unit=0  adc_ctu=off  adc_owr=on  adc_wls=Right  adc_clk=on  adc_ack=on  adc_ctr0_inp=off  adc_ctr0_shft=10 - Avin = 0  adc_ctr0_cmp=01  adc_ctr0_samp=4  adc_ctr1_inp=off  adc_ctr1_cmp=01  adc_ctr1_samp=1  adc_ctr1_tsens=PTAT  adc_pscr_preval=V0  adc_pscr_preconv=off
  Constant : Constant  Value=pot_offset  OutDataTypeStr=uint16
  Gain : Gain  Gain=pot_gain  OutDataTypeStr=float('single')
  Sum : Sum  Inputs=-+|  OutDataTypeStr=single
  Fd : Outport
  wires:
  Constant/1 -> Sum/1
  Sum/1 -> Gain/1
  Gain/1 -> Fd/1
  ADC Channel/1 -> Sum/2

== system Final_project/High Level Design/Inputs/get wheel position ==
  Counts to Radians : Subsystem
  eTimer CNTR Register Read : rappid_564xl_ec_toolbox/MPC564xL/Motor Control Blocks/eTimer CNTR Register Read  SubModule=0  TimerChan=0  subMod=0  channel=0
  Haptic Wheel Position (radians) : Outport
  wires:
  Counts to Radians/1(Radians) -> Haptic Wheel Position (radians)/1
  eTimer CNTR Register Read/1 -> Counts to Radians/1(Counts)

== system Final_project/High Level Design/Outputs/Extract x,y,psi ==
  s,n,psi,us : Inport
  Demux : Demux
  Mux : Mux  Inputs=3
  Terminator : Terminator
  s,n to x,y : Veh_Sim/s,n to x,y  SystemSampleTime=-1
  x,y,psi : Outport
  wires:
  Demux/1 -> s,n to x,y/1
  Demux/2 -> s,n to x,y/2
  s,n,psi,us/1 -> Demux/1
  s,n to x,y/1 -> Mux/1
  s,n to x,y/2 -> Mux/2
  Demux/3 -> Mux/3
  Mux/1 -> x,y,psi/1
  Demux/4 -> Terminator/1

== system Final_project/High Level Design/Outputs/Extract x,y,psi (Cars 1 - 6) ==
  s,n,psi,us (Cars 1 - 6) : Inport
  Demux : Demux  Outputs=6
  Extract x,y,psi : Subsystem
  Extract x,y,psi1 : Subsystem
  Extract x,y,psi2 : Subsystem
  Extract x,y,psi3 : Subsystem
  Extract x,y,psi4 : Subsystem
  Extract x,y,psi5 : Subsystem
  Mux : Mux  Inputs=6
  x,y,psi (Cars 1 - 6) : Outport
  wires:
  Demux/1 -> Extract x,y,psi/1(s,n,psi,us)
  Extract x,y,psi/1(x,y,psi) -> Mux/1
  Demux/2 -> Extract x,y,psi1/1(s,n,psi,us)
  Extract x,y,psi1/1(x,y,psi) -> Mux/2
  Demux/3 -> Extract x,y,psi2/1(s,n,psi,us)
  Extract x,y,psi2/1(x,y,psi) -> Mux/3
  Demux/4 -> Extract x,y,psi3/1(s,n,psi,us)
  Extract x,y,psi3/1(x,y,psi) -> Mux/4
  Demux/5 -> Extract x,y,psi4/1(s,n,psi,us)
  Extract x,y,psi4/1(x,y,psi) -> Mux/5
  s,n,psi,us (Cars 1 - 6)/1 -> Demux/1
  Mux/1 -> x,y,psi (Cars 1 - 6)/1
  Extract x,y,psi5/1(x,y,psi) -> Mux/6
  Demux/6 -> Extract x,y,psi5/1(s,n,psi,us)

== system Final_project/High Level Design/Outputs/Output s,n,psi,us ==
  s,n,psi.us : Inport
  CAN Transmit : rappid_564xl_ec_toolbox/MPC564xL/Communication Blocks/CAN Transmit  can_unit=A  can_unit_v2=0  can_buffer=0  can_id=45
  CAN Transmit2 : rappid_564xl_ec_toolbox/MPC564xL/Communication Blocks/CAN Transmit  can_unit=A  can_unit_v2=0  can_buffer=1  can_id=46
  Constant : Constant  Value=8  OutDataTypeStr=uint8
  Constant1 : Constant  Value=8  OutDataTypeStr=uint8
  Demux : Demux
  Mux1 : Mux  Inputs=2
  Mux2 : Mux  Inputs=2
  Single to Bytes{,1..3} (4 alike) : Conv_Lib/Single to Bytes
  wires:
  Single to Bytes/1 -> Mux1/1
  Single to Bytes1/1 -> Mux1/2
  Mux1/1 -> CAN Transmit/1
  Constant/1 -> CAN Transmit/2
  Mux2/1 -> CAN Transmit2/1
  Constant1/1 -> CAN Transmit2/2
  s,n,psi.us/1 -> Demux/1
  Demux/3 -> Single to Bytes2/1
  Demux/1 -> Single to Bytes/1
  Demux/4 -> Single to Bytes3/1
  Demux/2 -> Single to Bytes1/1
  Single to Bytes2/1 -> Mux2/2
  Single to Bytes3/1 -> Mux2/1

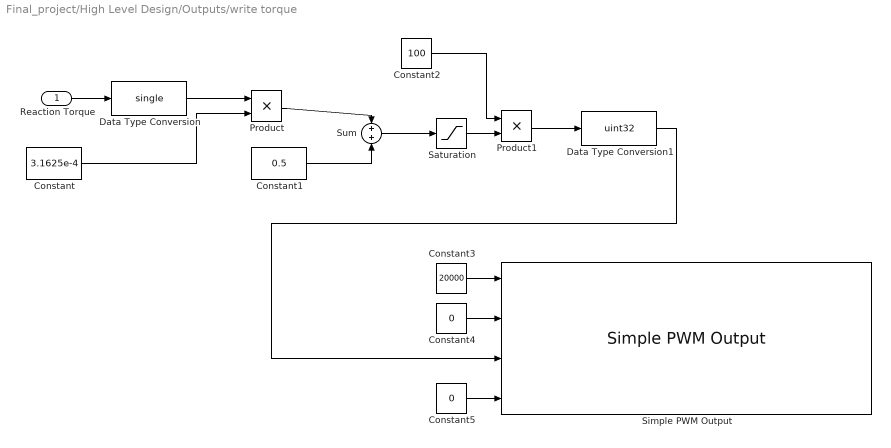
== system Final_project/High Level Design/Outputs/write torque ==
  Reaction Torque : Inport
  Constant : Constant  Value=3.1625e-4  OutDataTypeStr=single
  Constant1 : Constant  Value=0.5  OutDataTypeStr=single
  Constant2 : Constant  Value=100
  Constant3 : Constant  Value=20000  OutDataTypeStr=uint32
  Constant4 : Constant  Value=0  OutDataTypeStr=uint32
  Constant5 : Constant  Value=0  OutDataTypeStr=uint32
  Data Type Conversion : DataTypeConversion  OutDataTypeStr=single
  Data Type Conversion1 : DataTypeConversion  OutDataTypeStr=uint32
  Product : Product  RndMeth=Zero
  Product1 : Product  RndMeth=Zero
  Saturation : Saturate  UpperLimit=0.9  LowerLimit=0.1
  Simple PWM Output : rappid_564xl_ec_toolbox/MPC564xL/Motor Control Blocks/Simple PWM Output  Priority=1  pwmModule=0  pwmMod=0  SubModule=0  subMod=0  InitFreq=20000  resolution=1 %  resValue=1  InitDutyA=0  InitDutyB=50  align=A - edge aligned B - phase shifted  PhaseShift_A=0  PhaseShift=0  Phase_A=0  Phase_B=0  centered=-1  DoubleS=off  doubleSw=off  debugSw=off  debug_mode=0  pin_A0="58  : PD10 : [ 76 ] : [ T15 ]"  pin_B0="59  : PD11 : [ 78 ] : [ R16 ]"  pin_X0=None  pin_A1=None  pin_B1=None  pin_X1=None  pin_A2=None  pin_B2="100 : PG4  : [ 100 ] : [ F17 ]"  pin_X2=None  pin_A3=None  pin_B3=None  pin_X3=None  pin1_A0=None  pin1_B0=None  pin1_X0=None  pin1_A1=None  pin1_B1=None  pin1_X1=None  pin1_A2=None  pin1_B2=None  pin1_X2=None  pin1_A3=None  pin1_B3=None  pin1_X3=None  pcrNumA=58  pcrNumB=59  pcrNumX=255  polA=off  polB=off  polX=off  octrl=0  syncFrom0=off  masterSync=0  outVal0=off  outVal1=off  outVal2=on  outVal3=on  outVal4=on  outVal5=on  outTrig=60
  Sum : Sum  Inputs=+|+
  wires:
  Constant/1 -> Product/2
  Product/1 -> Sum/1
  Reaction Torque/1 -> Data Type Conversion/1
  Data Type Conversion/1 -> Product/1
  Constant1/1 -> Sum/2
  Sum/1 -> Saturation/1
  Saturation/1 -> Product1/2
  Constant2/1 -> Product1/1
  Product1/1 -> Data Type Conversion1/1
  Data Type Conversion1/1 -> Simple PWM Output/3
  Constant3/1 -> Simple PWM Output/1
  Constant4/1 -> Simple PWM Output/2
  Constant5/1 -> Simple PWM Output/4

== system Final_project/High Level Design/Automatic Cruise Control/Speed Ctrl/PI ==
  Error : Inport
  Gain : Gain  Gain=V_Ki  SaturateOnIntegerOverflow=on  OutDataTypeStr=Inherit: Same as input  ParamDataTypeStr=Inherit: Same as input
  Gain1 : Gain  Gain=V_Kp  SaturateOnIntegerOverflow=on  OutDataTypeStr=Inherit: Same as input  ParamDataTypeStr=Inherit: Same as input
  My Discrete Integrator : Subsystem
  Sum : Sum  Inputs=|++  SaturateOnIntegerOverflow=on
  U : Outport
  wires:
  Gain/1 -> My Discrete Integrator/1(X_dot)
  My Discrete Integrator/1(X) -> Sum/1
  Gain1/1 -> Sum/2
  Error/1 -> Gain/1, Gain1/1
  Sum/1 -> U/1

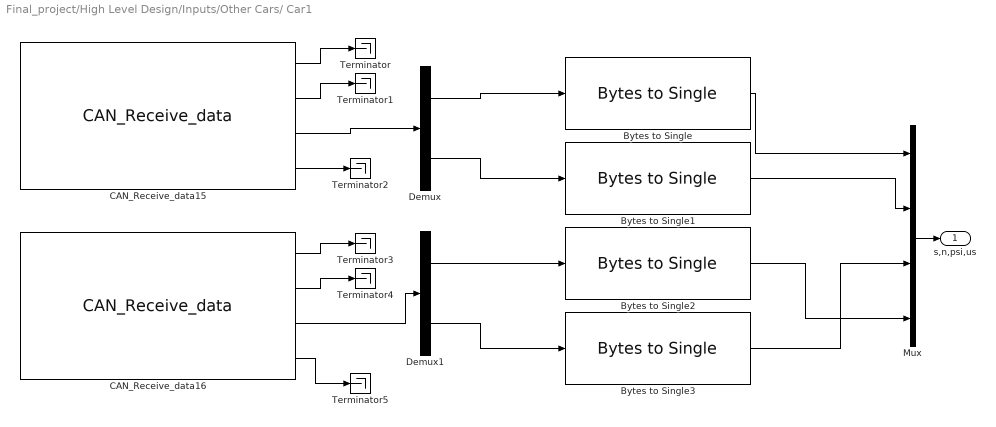
== system Final_project/High Level Design/Inputs/Other Cars/ Car1 ==
  Bytes to Single{,1..3} (4 alike) : Conv_Lib/Bytes to Single
  CAN_Receive_data15 : rappid_564xl_ec_toolbox/MPC564xL/Communication Blocks/CAN_Receive_data  can_unit=A  can_unit_v2=0  can_buffer=4  can_id=15
  CAN_Receive_data16 : rappid_564xl_ec_toolbox/MPC564xL/Communication Blocks/CAN_Receive_data  can_unit=A  can_unit_v2=0  can_buffer=5  can_id=16
  Demux : Demux  Outputs=2
  Demux1 : Demux  Outputs=2
  Mux : Mux
  Terminator{,1..5} (6 alike) : Terminator
  s,n,psi,us : Outport
  wires:
  Bytes to Single1/1 -> Mux/2
  Bytes to Single3/1 -> Mux/3
  Demux/1 -> Bytes to Single/1
  Demux/2 -> Bytes to Single1/1
  Demux1/1 -> Bytes to Single2/1
  Demux1/2 -> Bytes to Single3/1
  Bytes to Single/1 -> Mux/1
  Bytes to Single2/1 -> Mux/4
  Mux/1 -> s,n,psi,us/1
  CAN_Receive_data15/1 -> Terminator/1
  CAN_Receive_data15/2 -> Terminator1/1
  CAN_Receive_data15/3 -> Demux/1
  CAN_Receive_data15/4 -> Terminator2/1
  CAN_Receive_data16/1 -> Terminator3/1
  CAN_Receive_data16/2 -> Terminator4/1
  CAN_Receive_data16/3 -> Demux1/1
  CAN_Receive_data16/4 -> Terminator5/1

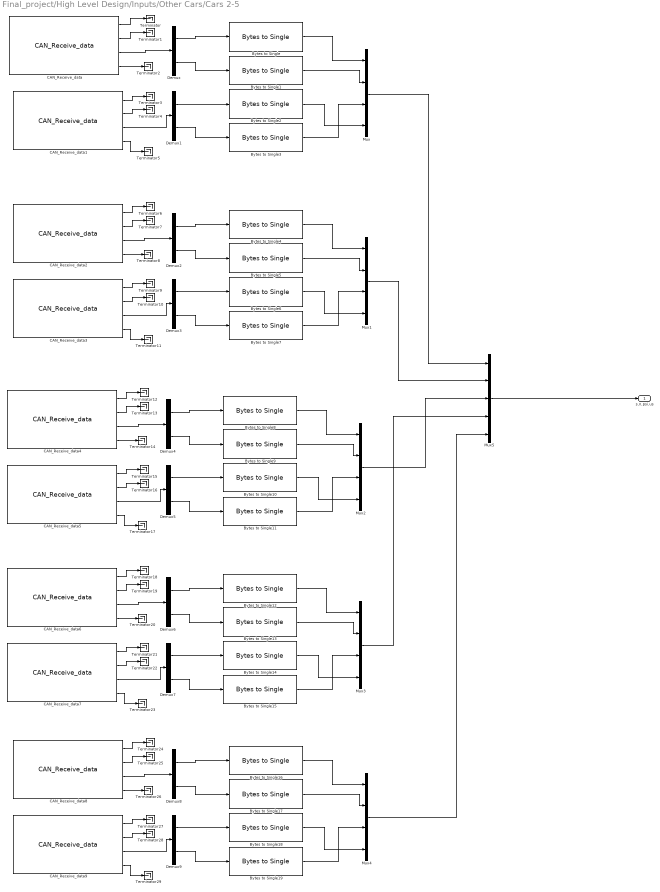
== system Final_project/High Level Design/Inputs/Other Cars/Cars 2-5 ==
  Bytes to Single{,1..19} (20 alike) : Conv_Lib/Bytes to Single
  CAN_Receive_data : rappid_564xl_ec_toolbox/MPC564xL/Communication Blocks/CAN_Receive_data  can_unit=A  can_unit_v2=0  can_buffer=6  can_id=25
  CAN_Receive_data1 : rappid_564xl_ec_toolbox/MPC564xL/Communication Blocks/CAN_Receive_data  can_unit=A  can_unit_v2=0  can_buffer=7  can_id=26
  CAN_Receive_data2 : rappid_564xl_ec_toolbox/MPC564xL/Communication Blocks/CAN_Receive_data  can_unit=A  can_unit_v2=0  can_buffer=8  can_id=35
  CAN_Receive_data3 : rappid_564xl_ec_toolbox/MPC564xL/Communication Blocks/CAN_Receive_data  can_unit=A  can_unit_v2=0  can_buffer=9  can_id=36
  CAN_Receive_data4 : rappid_564xl_ec_toolbox/MPC564xL/Communication Blocks/CAN_Receive_data  can_unit=A  can_unit_v2=0  can_buffer=10  can_id=75
  CAN_Receive_data5 : rappid_564xl_ec_toolbox/MPC564xL/Communication Blocks/CAN_Receive_data  can_unit=A  can_unit_v2=0  can_buffer=11  can_id=76
  CAN_Receive_data6 : rappid_564xl_ec_toolbox/MPC564xL/Communication Blocks/CAN_Receive_data  can_unit=A  can_unit_v2=0  can_buffer=12  can_id=65
  CAN_Receive_data7 : rappid_564xl_ec_toolbox/MPC564xL/Communication Blocks/CAN_Receive_data  can_unit=A  can_unit_v2=0  can_buffer=13  can_id=66
  CAN_Receive_data8 : rappid_564xl_ec_toolbox/MPC564xL/Communication Blocks/CAN_Receive_data  can_unit=A  can_unit_v2=0  can_buffer=14  can_id=55
  CAN_Receive_data9 : rappid_564xl_ec_toolbox/MPC564xL/Communication Blocks/CAN_Receive_data  can_unit=A  can_unit_v2=0  can_buffer=15  can_id=56
  Demux{,1..9} (10 alike) : Demux  Outputs=2
  Mux{,1..4} (5 alike) : Mux
  Mux5 : Mux  Inputs=5
  Terminator{,1..29} (30 alike) : Terminator
  s,n,psi,us : Outport
  wires:
  Bytes to Single1/1 -> Mux/2
  Bytes to Single3/1 -> Mux/3
  Demux/1 -> Bytes to Single/1
  Demux/2 -> Bytes to Single1/1
  Demux1/1 -> Bytes to Single2/1
  Demux1/2 -> Bytes to Single3/1
  Bytes to Single/1 -> Mux/1
  Bytes to Single2/1 -> Mux/4
  Mux/1 -> Mux5/1
  CAN_Receive_data/1 -> Terminator/1
  CAN_Receive_data/2 -> Terminator1/1
  CAN_Receive_data/3 -> Demux/1
  CAN_Receive_data/4 -> Terminator2/1
  CAN_Receive_data1/1 -> Terminator3/1
  CAN_Receive_data1/2 -> Terminator4/1
  CAN_Receive_data1/3 -> Demux1/1
  CAN_Receive_data1/4 -> Terminator5/1
  Bytes to Single5/1 -> Mux1/2
  Bytes to Single7/1 -> Mux1/3
  Demux2/1 -> Bytes to Single4/1
  Demux2/2 -> Bytes to Single5/1
  Demux3/1 -> Bytes to Single6/1
  Demux3/2 -> Bytes to Single7/1
  Bytes to Single4/1 -> Mux1/1
  Bytes to Single6/1 -> Mux1/4
  CAN_Receive_data2/1 -> Terminator6/1
  CAN_Receive_data2/2 -> Terminator7/1
  CAN_Receive_data2/3 -> Demux2/1
  CAN_Receive_data2/4 -> Terminator8/1
  CAN_Receive_data3/1 -> Terminator9/1
  CAN_Receive_data3/2 -> Terminator10/1
  CAN_Receive_data3/3 -> Demux3/1
  CAN_Receive_data3/4 -> Terminator11/1
  Bytes to Single9/1 -> Mux2/2
  Bytes to Single11/1 -> Mux2/3
  Demux4/1 -> Bytes to Single8/1
  Demux4/2 -> Bytes to Single9/1
  Demux5/1 -> Bytes to Single10/1
  Demux5/2 -> Bytes to Single11/1
  Bytes to Single8/1 -> Mux2/1
  Bytes to Single10/1 -> Mux2/4
  CAN_Receive_data4/1 -> Terminator12/1
  CAN_Receive_data4/2 -> Terminator13/1
  CAN_Receive_data4/3 -> Demux4/1
  CAN_Receive_data4/4 -> Terminator14/1
  CAN_Receive_data5/1 -> Terminator15/1
  CAN_Receive_data5/2 -> Terminator16/1
  CAN_Receive_data5/3 -> Demux5/1
  CAN_Receive_data5/4 -> Terminator17/1
  Bytes to Single13/1 -> Mux3/2
  Bytes to Single15/1 -> Mux3/3
  Demux6/1 -> Bytes to Single12/1
  Demux6/2 -> Bytes to Single13/1
  Demux7/1 -> Bytes to Single14/1
  Demux7/2 -> Bytes to Single15/1
  Bytes to Single12/1 -> Mux3/1
  Bytes to Single14/1 -> Mux3/4
  CAN_Receive_data6/1 -> Terminator18/1
  CAN_Receive_data6/2 -> Terminator19/1
  CAN_Receive_data6/3 -> Demux6/1
  CAN_Receive_data6/4 -> Terminator20/1
  CAN_Receive_data7/1 -> Terminator21/1
  CAN_Receive_data7/2 -> Terminator22/1
  CAN_Receive_data7/3 -> Demux7/1
  CAN_Receive_data7/4 -> Terminator23/1
  Bytes to Single17/1 -> Mux4/2
  Bytes to Single19/1 -> Mux4/3
  Demux8/1 -> Bytes to Single16/1
  Demux8/2 -> Bytes to Single17/1
  Demux9/1 -> Bytes to Single18/1
  Demux9/2 -> Bytes to Single19/1
  Bytes to Single16/1 -> Mux4/1
  Bytes to Single18/1 -> Mux4/4
  Mux4/1 -> Mux5/5
  CAN_Receive_data8/1 -> Terminator24/1
  CAN_Receive_data8/2 -> Terminator25/1
  CAN_Receive_data8/3 -> Demux8/1
  CAN_Receive_data8/4 -> Terminator26/1
  CAN_Receive_data9/1 -> Terminator27/1
  CAN_Receive_data9/2 -> Terminator28/1
  CAN_Receive_data9/3 -> Demux9/1
  CAN_Receive_data9/4 -> Terminator29/1
  Mux5/1 -> s,n,psi,us/1
  Mux1/1 -> Mux5/2
  Mux2/1 -> Mux5/3
  Mux3/1 -> Mux5/4

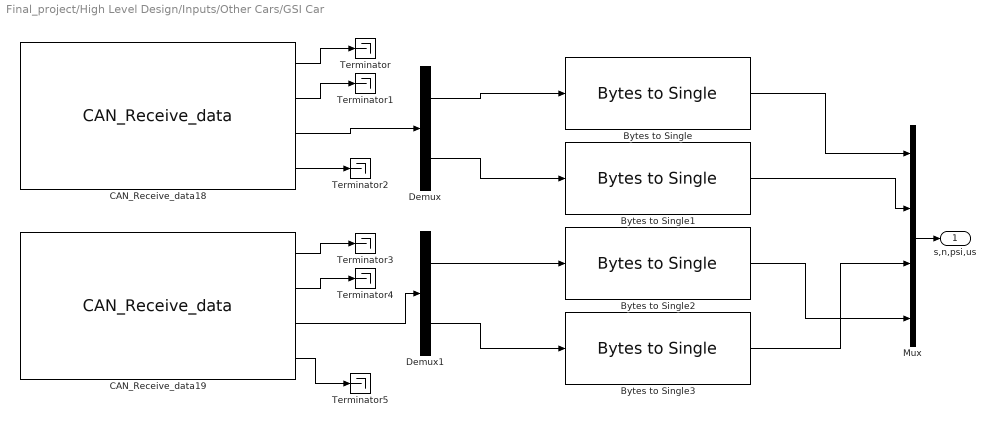
== system Final_project/High Level Design/Inputs/Other Cars/GSI Car ==
  Bytes to Single{,1..3} (4 alike) : Conv_Lib/Bytes to Single
  CAN_Receive_data18 : rappid_564xl_ec_toolbox/MPC564xL/Communication Blocks/CAN_Receive_data  can_unit=A  can_unit_v2=0  can_buffer=2  can_id=105
  CAN_Receive_data19 : rappid_564xl_ec_toolbox/MPC564xL/Communication Blocks/CAN_Receive_data  can_unit=A  can_unit_v2=0  can_buffer=3  can_id=106
  Demux : Demux  Outputs=2
  Demux1 : Demux  Outputs=2
  Mux : Mux
  Terminator{,1..5} (6 alike) : Terminator
  s,n,psi,us : Outport
  wires:
  Bytes to Single1/1 -> Mux/2
  Bytes to Single3/1 -> Mux/3
  Demux/1 -> Bytes to Single/1
  Demux/2 -> Bytes to Single1/1
  Demux1/1 -> Bytes to Single2/1
  Demux1/2 -> Bytes to Single3/1
  Bytes to Single/1 -> Mux/1
  Bytes to Single2/1 -> Mux/4
  Mux/1 -> s,n,psi,us/1
  CAN_Receive_data18/1 -> Terminator/1
  CAN_Receive_data18/2 -> Terminator1/1
  CAN_Receive_data18/3 -> Demux/1
  CAN_Receive_data18/4 -> Terminator2/1
  CAN_Receive_data19/1 -> Terminator3/1
  CAN_Receive_data19/2 -> Terminator4/1
  CAN_Receive_data19/3 -> Demux1/1
  CAN_Receive_data19/4 -> Terminator5/1

== system Final_project/High Level Design/Inputs/Other Cars/Zeros (16) ==
  Constant : Constant  Value=0  OutDataTypeStr=single
  Mux : Mux  Inputs=20
  Zeros : Outport
  wires:
  Constant/1 -> Mux/1, Mux/2, Mux/3, Mux/4, Mux/5, Mux/6, Mux/7, Mux/8, Mux/9, Mux/10, Mux/11, Mux/12, Mux/16, Mux/13, Mux/19, Mux/20, Mux/15, Mux/18, Mux/14, Mux/17
  Mux/1 -> Zeros/1

== system Final_project/High Level Design/Inputs/get wheel position/Counts to Radians ==
  Counts : Inport
  Data Type Conversion : DataTypeConversion  OutDataTypeStr=uint16
  Data Type Conversion1 : DataTypeConversion  OutDataTypeStr=int16
  Data Type Conversion2 : DataTypeConversion  OutDataTypeStr=single
  Delay : Delay  DelayLength=1
  Delay1 : Delay  DelayLength=1
  Gain : Gain  Gain=-2*pi()/4000  OutDataTypeStr=single
  Sum : Sum  Inputs=|+-
  Sum1 : Sum  Inputs=|++
  Radians : Outport
  wires:
  Data Type Conversion/1 -> Sum/1, Delay/1
  Delay/1 -> Sum/2
  Sum1/1 -> Delay1/1, Radians/1
  Delay1/1 -> Sum1/2
  Gain/1 -> Sum1/1
  Data Type Conversion2/1 -> Gain/1
  Data Type Conversion1/1 -> Data Type Conversion2/1
  Sum/1 -> Data Type Conversion1/1
  Counts/1 -> Data Type Conversion/1

== system Final_project/High Level Design/Outputs/Extract x,y,psi (Cars 1 - 6)/Extract x,y,psi ==
  s,n,psi,us : Inport
  Demux : Demux
  Mux : Mux  Inputs=3
  Terminator : Terminator
  s,n to x,y : Veh_Sim/s,n to x,y  SystemSampleTime=-1
  x,y,psi : Outport
  wires:
  Demux/1 -> s,n to x,y/1
  Demux/2 -> s,n to x,y/2
  s,n,psi,us/1 -> Demux/1
  s,n to x,y/1 -> Mux/1
  s,n to x,y/2 -> Mux/2
  Demux/3 -> Mux/3
  Mux/1 -> x,y,psi/1
  Demux/4 -> Terminator/1

== system Final_project/High Level Design/Outputs/Extract x,y,psi (Cars 1 - 6)/Extract x,y,psi1 ==
  s,n,psi,us : Inport
  Demux : Demux
  Mux : Mux  Inputs=3
  Terminator : Terminator
  s,n to x,y : Veh_Sim/s,n to x,y  SystemSampleTime=-1
  x,y,psi : Outport
  wires:
  Demux/1 -> s,n to x,y/1
  Demux/2 -> s,n to x,y/2
  s,n,psi,us/1 -> Demux/1
  s,n to x,y/1 -> Mux/1
  s,n to x,y/2 -> Mux/2
  Demux/3 -> Mux/3
  Mux/1 -> x,y,psi/1
  Demux/4 -> Terminator/1

== system Final_project/High Level Design/Outputs/Extract x,y,psi (Cars 1 - 6)/Extract x,y,psi2 ==
  s,n,psi,us : Inport
  Demux : Demux
  Mux : Mux  Inputs=3
  Terminator : Terminator
  s,n to x,y : Veh_Sim/s,n to x,y  SystemSampleTime=-1
  x,y,psi : Outport
  wires:
  Demux/1 -> s,n to x,y/1
  Demux/2 -> s,n to x,y/2
  s,n,psi,us/1 -> Demux/1
  s,n to x,y/1 -> Mux/1
  s,n to x,y/2 -> Mux/2
  Demux/3 -> Mux/3
  Mux/1 -> x,y,psi/1
  Demux/4 -> Terminator/1

== system Final_project/High Level Design/Outputs/Extract x,y,psi (Cars 1 - 6)/Extract x,y,psi3 ==
  s,n,psi,us : Inport
  Demux : Demux
  Mux : Mux  Inputs=3
  Terminator : Terminator
  s,n to x,y : Veh_Sim/s,n to x,y  SystemSampleTime=-1
  x,y,psi : Outport
  wires:
  Demux/1 -> s,n to x,y/1
  Demux/2 -> s,n to x,y/2
  s,n,psi,us/1 -> Demux/1
  s,n to x,y/1 -> Mux/1
  s,n to x,y/2 -> Mux/2
  Demux/3 -> Mux/3
  Mux/1 -> x,y,psi/1
  Demux/4 -> Terminator/1

== system Final_project/High Level Design/Outputs/Extract x,y,psi (Cars 1 - 6)/Extract x,y,psi4 ==
  s,n,psi,us : Inport
  Demux : Demux
  Mux : Mux  Inputs=3
  Terminator : Terminator
  s,n to x,y : Veh_Sim/s,n to x,y  SystemSampleTime=-1
  x,y,psi : Outport
  wires:
  Demux/1 -> s,n to x,y/1
  Demux/2 -> s,n to x,y/2
  s,n,psi,us/1 -> Demux/1
  s,n to x,y/1 -> Mux/1
  s,n to x,y/2 -> Mux/2
  Demux/3 -> Mux/3
  Mux/1 -> x,y,psi/1
  Demux/4 -> Terminator/1

== system Final_project/High Level Design/Outputs/Extract x,y,psi (Cars 1 - 6)/Extract x,y,psi5 ==
  s,n,psi,us : Inport
  Demux : Demux
  Mux : Mux  Inputs=3
  Terminator : Terminator
  s,n to x,y : Veh_Sim/s,n to x,y  SystemSampleTime=-1
  x,y,psi : Outport
  wires:
  Demux/1 -> s,n to x,y/1
  Demux/2 -> s,n to x,y/2
  s,n,psi,us/1 -> Demux/1
  s,n to x,y/1 -> Mux/1
  s,n to x,y/2 -> Mux/2
  Demux/3 -> Mux/3
  Mux/1 -> x,y,psi/1
  Demux/4 -> Terminator/1
